simulink model "engineuntitled"  (R2025b)
settings: Solver=ode15s  StartTime=0.0  StopTime=15  FixedStep=1e-5  MaxStep=1e-4  MinStep=1e-10  RelTol=1e-5  AbsTol=1e-5
undefined symbols (not defined in the file or in its folder): constantsSTADPOLE
settings Model: Creator=alex2  LastModifiedBy=alex2
settings SolverCC: AutoScaleAbsTol=off  InitialStep=1e-9  MaxOrder=4.0

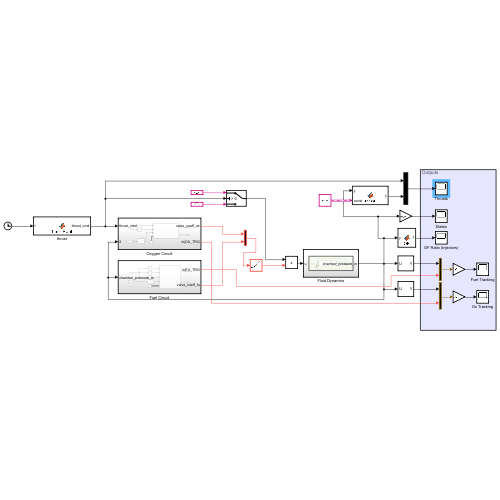
[thumbnail: Simulink's stored preview of the top-level diagram]
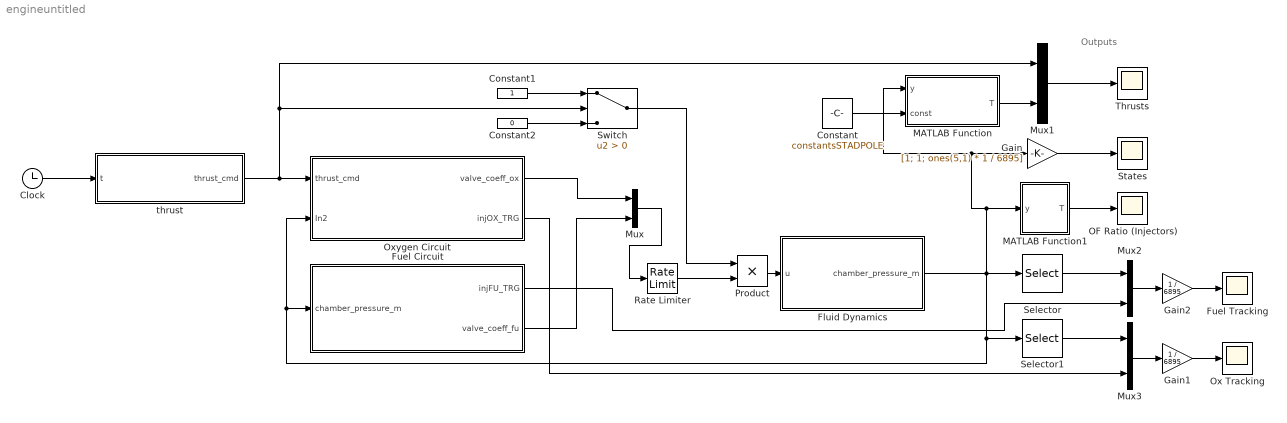
== system engineuntitled ==
  note: Outputs
  Clock : Clock
  Constant : Constant  Value=constantsSTADPOLE  OutDataTypeStr=Bus: slBus1
  Constant1 : Constant
  Constant2 : Constant  Value=0
  Fluid Dynamics : Subsystem
  Fuel Circuit : Subsystem
  Fuel Tracking : Scope
      settings: ActiveDisplayYMinimum=-65.371511244894648  ActiveDisplayYMaximum=503.93015589534451  DataLoggingVariableName=ScopeData3
  Gain : Gain  Gain=[1; 1; ones(5,1) * 1 / 6895]
  Gain1 : Gain  Gain=1 / 6895
  Gain2 : Gain  Gain=1 / 6895
  MATLAB Function : MATLAB Function  TreatAsAtomicUnit=on
  MATLAB Function1 : MATLAB Function  TreatAsAtomicUnit=on
  Mux{,1..3} (4 alike) : Mux  Inputs=2
  OF Ratio (Injectors) : Scope
      settings: ActiveDisplayYMinimum=0  ActiveDisplayYMaximum=3  DataLoggingVariableName=ScopeData2
  Ox Tracking : Scope
      settings: ActiveDisplayYMinimum=-52.544225777854543  ActiveDisplayYMaximum=458.85039791193037  DataLoggingVariableName=ScopeData4
  Oxygen Circuit : Subsystem
  Product : Product
  Rate Limiter : RateLimiter  RisingSlewLimit=10^-4  FallingSlewLimit=-10^-4  SampleTimeMode=inherited
  Selector : Selector  IndexOptions=Index vector (dialog)  Indices=5  OutputSizes=1
  Selector1 : Selector  IndexOptions=Index vector (dialog)  Indices=4  OutputSizes=1
  States : Scope
      settings: ActiveDisplayYMinimum=-5.4008603558354062E+12  ActiveDisplayYMaximum=4.8586415626429461E+13
  Switch : Switch  Criteria=u2 > Threshold  SaturateOnIntegerOverflow=off  InputSameDT=off
  Thrusts : Scope
      settings: ActiveDisplayYMinimum=568.03096239670776  ActiveDisplayYMaximum=2441.1065101836757
  thrust : MATLAB Function  TreatAsAtomicUnit=on
  wires:
  Clock/1 -> thrust/1(t)
  thrust/1(thrust_cmd) -> Mux1/1, Switch/2, Oxygen Circuit/1(thrust_cmd)
  MATLAB Function/1(T) -> Mux1/2
  Constant/1 -> MATLAB Function/2(const)
  Mux1/1 -> Thrusts/1
  MATLAB Function1/1(T) -> OF Ratio (Injectors)/1
  Gain/1 -> States/1
  Mux/1 -> Rate Limiter/1
  Rate Limiter/1 -> Product/2
  Product/1 -> Fluid Dynamics/1(u)
  Switch/1 -> Product/1
  Constant1/1 -> Switch/1
  Constant2/1 -> Switch/3
  Mux2/1 -> Gain2/1
  Selector/1 -> Mux2/1
  Mux3/1 -> Gain1/1
  Selector1/1 -> Mux3/1
  Gain1/1 -> Ox Tracking/1
  Gain2/1 -> Fuel Tracking/1
  Fluid Dynamics/1(chamber_pressure_m) -> Fuel Circuit/1(chamber_pressure_m), Oxygen Circuit/2(In2), Selector1/1, Selector/1, MATLAB Function1/1(y), Gain/1, MATLAB Function/1(y)
  Oxygen Circuit/1(valve_coeff_ox) -> Mux/1
  Fuel Circuit/2(valve_coeff_fu) -> Mux/2
  Oxygen Circuit/2(injOX_TRG) -> Mux3/2
  Fuel Circuit/1(injFU_TRG) -> Mux2/2

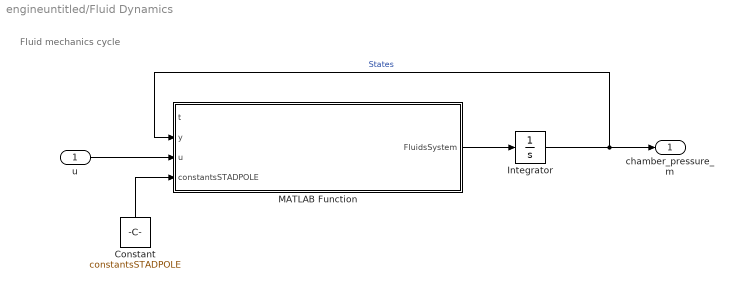
== system engineuntitled/Fluid Dynamics ==
  note: Fluid mechanics cycle
  u : Inport
  Constant : Constant  Value=constantsSTADPOLE  OutDataTypeStr=Bus: slBus1
  Integrator : Integrator  InitialCondition=constantsSTADPOLE.init_cond
  MATLAB Function : MATLAB Function  TreatAsAtomicUnit=on
  chamber_pressure_m : Outport
  wires:
  Integrator/1 -> chamber_pressure_m/1, MATLAB Function/2(y)  "States"
  MATLAB Function/1(FluidsSystem) -> Integrator/1
  Constant/1 -> MATLAB Function/4(constantsSTADPOLE)
  u/1 -> MATLAB Function/3(u)

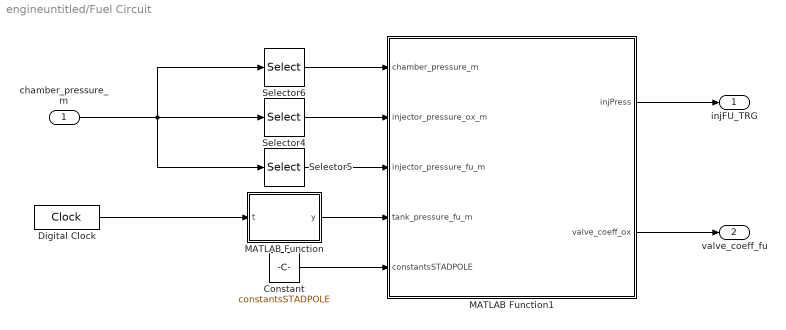
== system engineuntitled/Fuel Circuit ==
  chamber_pressure_m : Inport
  Constant : Constant  Value=constantsSTADPOLE  OutDataTypeStr=Bus: slBus1
  Digital Clock : DigitalClock  SampleTime=1e-4
  MATLAB Function : MATLAB Function  TreatAsAtomicUnit=on
  MATLAB Function1 : MATLAB Function  TreatAsAtomicUnit=on
  Selector4 : Selector  InputPortWidth=7  IndexOptions=Index vector (dialog)  Indices=4  OutputSizes=1
  Selector5 : Selector  InputPortWidth=7  IndexOptions=Index vector (dialog)  Indices=5  OutputSizes=1
  Selector6 : Selector  InputPortWidth=7  IndexOptions=Index vector (dialog)  Indices=3  OutputSizes=1
  injFU_TRG : Outport
  valve_coeff_fu : Outport  Port=2
  wires:
  Constant/1 -> MATLAB Function1/5(constantsSTADPOLE)
  chamber_pressure_m/1 -> Selector6/1, Selector4/1, Selector5/1
  MATLAB Function/1(y) -> MATLAB Function1/4(tank_pressure_fu_m)
  Digital Clock/1 -> MATLAB Function/1(t)
  Selector4/1 -> MATLAB Function1/2(injector_pressure_ox_m)
  Selector5/1 -> MATLAB Function1/3(injector_pressure_fu_m)
  Selector6/1 -> MATLAB Function1/1(chamber_pressure_m)
  MATLAB Function1/1(injPress) -> injFU_TRG/1
  MATLAB Function1/2(valve_coeff_ox) -> valve_coeff_fu/1

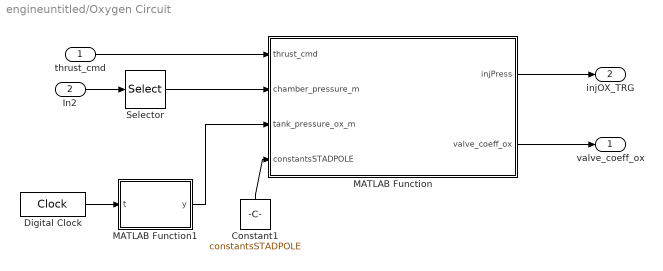
== system engineuntitled/Oxygen Circuit ==
  thrust_cmd : Inport
  In2 : Inport  Port=2
  Constant1 : Constant  Value=constantsSTADPOLE  OutDataTypeStr=Bus: slBus1
  Digital Clock : DigitalClock  SampleTime=1e-4
  MATLAB Function : MATLAB Function  TreatAsAtomicUnit=on
  MATLAB Function1 : MATLAB Function  TreatAsAtomicUnit=on
  Selector : Selector  InputPortWidth=7  IndexOptions=Index vector (dialog)  Indices=3  OutputSizes=1
  valve_coeff_ox : Outport
  injOX_TRG : Outport  Port=2
  wires:
  Constant1/1 -> MATLAB Function/4(constantsSTADPOLE)
  thrust_cmd/1 -> MATLAB Function/1(thrust_cmd)
  In2/1 -> Selector/1
  Selector/1 -> MATLAB Function/2(chamber_pressure_m)
  MATLAB Function1/1(y) -> MATLAB Function/3(tank_pressure_ox_m)
  Digital Clock/1 -> MATLAB Function1/1(t)
  MATLAB Function/1(injPress) -> injOX_TRG/1
  MATLAB Function/2(valve_coeff_ox) -> valve_coeff_ox/1

== matlab function engineuntitled/Fluid Dynamics/MATLAB Function ==
  data: t input; FluidsSystem output; y input; u input; constantsSTADPOLE input
function FluidsSystem = fluidMechanics(t, y, u, constantsSTADPOLE)
    
    % y(1)' = time rate of mass flow oxygen [kg/s^2]
    % y(2)' = time rate of mass flow fuel [kg/s^2]
    % y(3)' = time rate of chamber pressure [Pa/s]
    % y(4)' = time rate of oxygen injector press [Pa/s]
    % y(5)' = time rate of fuel injector press [Pa/s]
    % y(6)' = time rate of oxygen pressure at valve [Pa/s]
    % y(7)' = time rate of fuel pressure at valve [Pa/s]

    % y(1) = mass flow oxygen across pipe [kg/s]
    % y(2) = mass flow fuel across pipe [kg/s]
    % y(3) = chamber pressure [Pa]
    % y(4) = oxygen pressure at inj [Pa]
    % y(5) = fuel pressure at inj [Pa]
    % y(6) = oxygen pressure at valve [Pa]
    % y(7) = fuel pressure at valve [Pa]
    
    a_t= constantsSTADPOLE.a_t ; % [m^2], throat area
    
    dens_o = constantsSTADPOLE.dens_o; % [kg/m^3], liquid oxygen density, at 90 K and 1 atm
    dens_f = constantsSTADPOLE.dens_f ; % [kg/m^3], fuel density, at 293 K and 1 atm
    dens_w = constantsSTADPOLE.dens_w ; % [kg/m^3], water density
    g = constantsSTADPOLE.g ; % [m/s^2], acceleration due to gravity
    a_i_o = constantsSTADPOLE.a_i_o; % [m^2] area injector ox
    a_i_f = constantsSTADPOLE.a_i_f ; % [m^2] area injector fuel
    r = constantsSTADPOLE.r ; % [J/kg-K], specific gas constant of exhaust (molecular weight 18.8 g/mol)
    c_star = constantsSTADPOLE.c_star ; % [m/s] characteristic velocity
    of = constantsSTADPOLE.OF_target;

    c_fric = 0.03; % [unitless], line friction coefficient
    c_d_o = constantsSTADPOLE.d_coeff_ox; % [unitless], oxygen injector coefficient
    c_d_f = constantsSTADPOLE.d_coeff_fu; % [unitless], fuel injector coefficient
    l_eq_o = 7 * 0.0254; % [m], oxygen equivalent line length 
    l_eq_f = 7 * 0.0254; % [m], fuel equivalent line length 
    l_o = 120 * 0.0254; % [m], oxygen line length
    l_f = 60 * 0.0254; % [m], fuel line length
    d = (0.5 - 2 * 0.065) * 0.0254; % [m], line diameter
    v_c = 1.103170594 * 1e-3; % [m^3], chamber volume
    a_l = pi * (d / 2) ^ 2; % [m^2], line area
  
    v_l_o = a_l * l_o;
    v_l_f = a_l * l_f;
    t_o = 90; 
    t_f = 293;

    % Assume constant?
    c_v_o = AngleToCoefficient(u(1,1)) %1.231e-06; % [m^3.5/kg^0.5], oxygen valve coefficient
    c_v_f = AngleToCoefficient(u(2,1)); %1.231e-06; % [], fuel valve coefficient
    p_tank_o = 3.792E6; % [Pa]
    p_tank_f = 3.792E6; % [Pa]
    t_c = 3570; % [K], chamber temperature
    

    del_p_i_o = 1 / (2 * dens_o * (c_d_o * a_i_o) ^ 2); 
    del_p_l_o = 96402.2;
    del_p_i_f = 1 / (2 * dens_f * (c_d_f * a_i_f) ^ 2); 
    del_p_l_f = 2082581.1;
    

    % Momentum equations
    % massflow across pipe
    % mdot_pipe_ox = (y(4) - y(3) - del_p_l_o * y(1) * sqrt(y(1)^2 + 1e-6)) * a_l / l_o;
    % mdot_pipe_fu = (y(5) - y(3) - del_p_l_f * y(2) * sqrt(y(2)^2 + 1e-6)) * a_l / l_f;
    mddot_pipe_ox = (y(6) - y(4) - del_p_l_o * y(1) * sqrt(y(1)^2 + 1e-6)) * a_l / l_o;
    mddot_pipe_fu = (y(7) - y(5) - del_p_l_f * y(2) * sqrt(y(2)^2 + 1e-6)) * a_l / l_f;

    % Valve massflows
    ValveOX = dens_o * dens_w * (p_tank_o - y(6));
    ValveFU = dens_f * dens_w * (p_tank_f - y(7));
    mdot_valve_ox = c_v_o * ValveOX / sqrt(abs(ValveOX) + 1e2);
    mdot_valve_fu = c_v_f * ValveFU / sqrt(abs(ValveFU) + 1e2);

    % Injector massflows
    InjectorOX = 2 * dens_o *(y(4)-y(3));
    InjectorFU = 2 * dens_f * (y(5)-y(3));
    mdot_inj_ox = c_d_o * a_i_o * InjectorOX / sqrt(abs(InjectorOX)+1e2);
    mdot_inj_fu = c_d_f * a_i_f * InjectorFU / sqrt(abs(InjectorFU)+1e2);

    % Pressure at the end of the valve
    valve_ox_dot = 1e9 / (v_l_o * dens_o) * (mdot_valve_ox - y(1));
    valve_fu_dot = 1e9 / (v_l_f * dens_f) * (mdot_valve_fu - y(2));

    inj_ox_dot = 1e9 / (v_l_o*dens_o) * (y(1) - mdot_inj_ox);
    inj_fu_dot = 1e9 / (v_l_f*dens_f) * (y(2) - mdot_inj_fu);

    % Chamber Pressure equations
    pdot_chamber = (r * t_c / v_c) * (mdot_inj_ox + mdot_inj_fu - a_t * y(3) / c_star);

    % Final system
    FluidsSystem = [mddot_pipe_ox; mddot_pipe_fu; pdot_chamber; inj_ox_dot; inj_fu_dot; valve_ox_dot; valve_fu_dot];
end

== matlab function engineuntitled/thrust ==
  data: t input; thrust_cmd output
function thrust_cmd = ThrustPlant(t)
%THRUSTPLANT 
%   random plant function for the thrust in the engine
if t < 2
    thrust_cmd = 0; %[N]
elseif mod(t,5) < 3
    thrust_cmd = 1500;
else
    thrust_cmd = 1500 - 500 * sin(mod(t,5) * pi / 2);
    
end
%cosint(t*pi/180);

end

== matlab function engineuntitled/Oxygen Circuit/MATLAB Function ==
  settings: updateMethod=DISCRETE
  data: injPress output; valve_coeff_ox output; thrust_cmd input; chamber_pressure_m input; tank_pressure_ox_m input; constantsSTADPOLE input
function [injPress, valve_coeff_ox] = leadValveOx(thrust_cmd, chamber_pressure_m, tank_pressure_ox_m, constantsSTADPOLE)
% Oxygen circuit code
[injPress, valve_coeff_ox] = oxygenCircuit(thrust_cmd, chamber_pressure_m, tank_pressure_ox_m, constantsSTADPOLE);

== matlab function engineuntitled/Fuel Circuit/MATLAB Function1 ==
  settings: updateMethod=DISCRETE
  data: injPress output; chamber_pressure_m input; injector_pressure_ox_m input; injector_pressure_fu_m input; tank_pressure_fu_m input; constantsSTADPOLE input; valve_coeff_ox output
function [injPress, valve_coeff_ox] = followValveFu(chamber_pressure_m, injector_pressure_ox_m, injector_pressure_fu_m, tank_pressure_fu_m, constantsSTADPOLE)

% Fuel circuit code
[injPress, valve_coeff_ox] = fuelCircuit(chamber_pressure_m, injector_pressure_ox_m, injector_pressure_fu_m, tank_pressure_fu_m, constantsSTADPOLE);

== matlab function engineuntitled/Oxygen Circuit/MATLAB Function1 ==
  data: t input; y output
function y = fcn(t)

% Simulate oxygen tank pressure, for now, assume constant at 5 MPa
y = 3.792E6; % [MPa]

== matlab function engineuntitled/Fuel Circuit/MATLAB Function ==
  data: t input; y output
function y = fcn(t)

% Simulate fuel tank pressure, for now, assume constant at 550 psi or 3.79
% MPa
% added small noise
y = 3.792E6; % [Pa]

== matlab function engineuntitled/MATLAB Function ==
  data: y input; T output; const input
function T = thrust(y, const)

T = y(3) * const.c_f * const.a_t;

== matlab function engineuntitled/MATLAB Function1 ==
  data: y input; T output
function T = OF(y)

T = y(1) / y(2);
